simulink model "FunnyScript"  (R2022b)
settings: Solver=VariableStepAuto  StartTime=0.0  StopTime=10.0  RelTol=1e-3
settings Model: Creator=tilog  LastModifiedBy=tilog

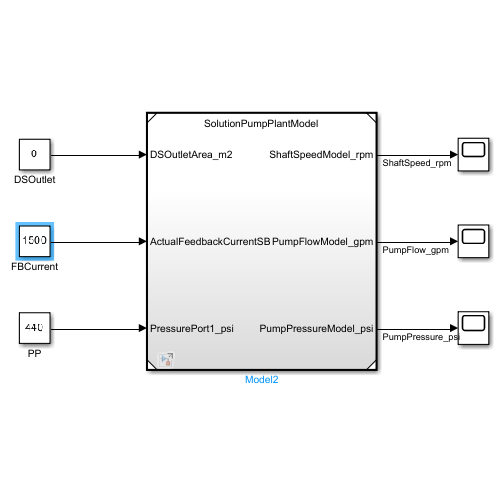
[thumbnail: Simulink's stored preview of the top-level diagram]
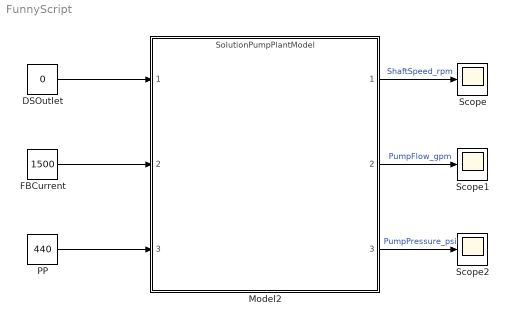
== system FunnyScript ==
  DSOutlet : Constant  Value=0
  FBCurrent : Constant  Value=1500
  Model2 : ModelReference  ModelNameDialog=SolutionPumpPlantModel.slx  SimulationMode=Normal  ModelReferenceVersion=1.2
  PP : Constant  Value=440
  Scope : Scope
  Scope1 : Scope
  Scope2 : Scope
  wires:
  DSOutlet/1 -> Model2/1
  PP/1 -> Model2/3
  FBCurrent/1 -> Model2/2
  Model2/3 -> Scope2/1  "PumpPressure_psi"
  Model2/2 -> Scope1/1  "PumpFlow_gpm"
  Model2/1 -> Scope/1  "ShaftSpeed_rpm"
